simulink model "ME131_lab8"  (R2018b)
settings: Solver=VariableStepAuto  StartTime=0.0  StopTime=29  RelTol=1e-3
undefined symbols (not defined in the file): Cf, Cr, dt, Iz, Lf, Lr, m, Vx0, Vy0, X0, Y0, yaw0, yawRate0
settings Model: Creator=YW_Liao  LastModifiedBy=trey
settings SFSimCC: SimUseLocalCustomCode=off
settings RTWCC: RTWUseLocalCustomCode=off

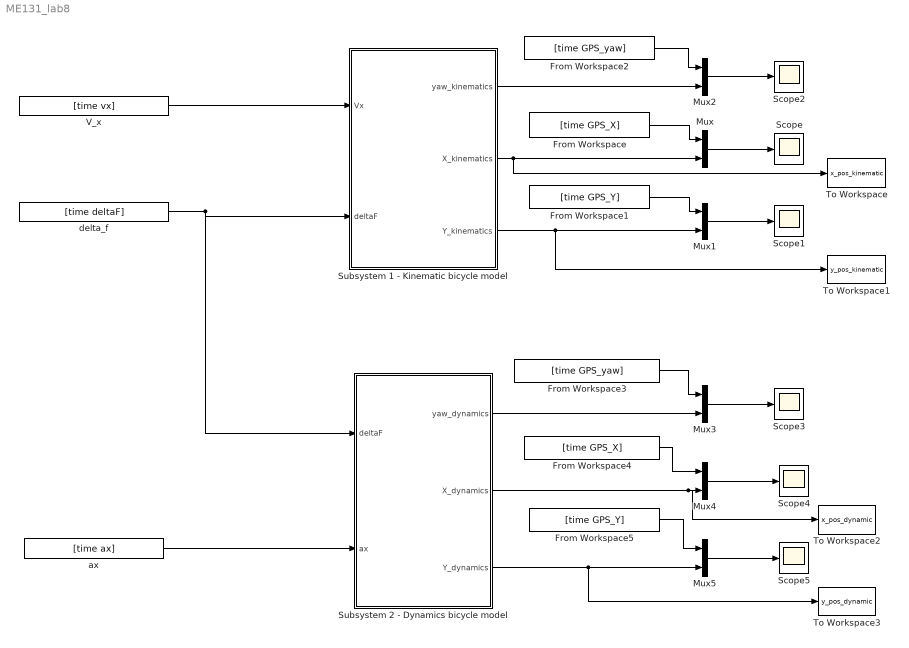
== system ME131_lab8 ==
  From Workspace : FromWorkspace  VariableName=[time GPS_X]  SampleTime=dt
  From Workspace1 : FromWorkspace  VariableName=[time GPS_Y]  SampleTime=dt
  From Workspace2 : FromWorkspace  VariableName=[time GPS_yaw]  SampleTime=dt
  From Workspace3 : FromWorkspace  VariableName=[time GPS_yaw]  SampleTime=dt
  From Workspace4 : FromWorkspace  VariableName=[time GPS_X]  SampleTime=dt
  From Workspace5 : FromWorkspace  VariableName=[time GPS_Y]  SampleTime=dt
  Mux{,1..5} (6 alike) : Mux  Inputs=2
  Scope{,1..5} (6 alike) : Scope
  Subsystem 1 - Kinematic bicycle model : Subsystem
  Subsystem 2 - Dynamics bicycle model : Subsystem
  To Workspace : ToWorkspace  VariableName=x_pos_kinematic  SaveFormat=Timeseries  SampleTime=-1
  To Workspace1 : ToWorkspace  VariableName=y_pos_kinematic  SaveFormat=Timeseries  SampleTime=-1
  To Workspace2 : ToWorkspace  VariableName=x_pos_dynamic  SaveFormat=Timeseries  SampleTime=-1
  To Workspace3 : ToWorkspace  VariableName=y_pos_dynamic  SaveFormat=Timeseries  SampleTime=-1
  V_x : FromWorkspace  VariableName=[time vx]  SampleTime=dt
  ax : FromWorkspace  VariableName=[time ax]  SampleTime=dt
  delta_f : FromWorkspace  VariableName=[time deltaF]  SampleTime=dt
  wires:
  Mux1/1 -> Scope1/1
  Mux/1 -> Scope/1
  From Workspace/1 -> Mux/1
  From Workspace1/1 -> Mux1/1
  Mux2/1 -> Scope2/1
  From Workspace2/1 -> Mux2/1
  From Workspace4/1 -> Mux4/1
  From Workspace3/1 -> Mux3/1
  Mux3/1 -> Scope3/1
  Mux4/1 -> Scope4/1
  Mux5/1 -> Scope5/1
  From Workspace5/1 -> Mux5/1
  Subsystem 1 - Kinematic bicycle model/3(Y_kinematics) -> To Workspace1/1, Mux1/2
  Subsystem 1 - Kinematic bicycle model/2(X_kinematics) -> To Workspace/1, Mux/2
  V_x/1 -> Subsystem 1 - Kinematic bicycle model/1(Vx)
  delta_f/1 -> Subsystem 2 - Dynamics bicycle model/1(deltaF), Subsystem 1 - Kinematic bicycle model/2(deltaF)
  Subsystem 1 - Kinematic bicycle model/1(yaw_kinematics) -> Mux2/2
  ax/1 -> Subsystem 2 - Dynamics bicycle model/2(ax)
  Subsystem 2 - Dynamics bicycle model/1(yaw_dynamics) -> Mux3/2
  Subsystem 2 - Dynamics bicycle model/2(X_dynamics) -> To Workspace2/1, Mux4/2
  Subsystem 2 - Dynamics bicycle model/3(Y_dynamics) -> To Workspace3/1, Mux5/2

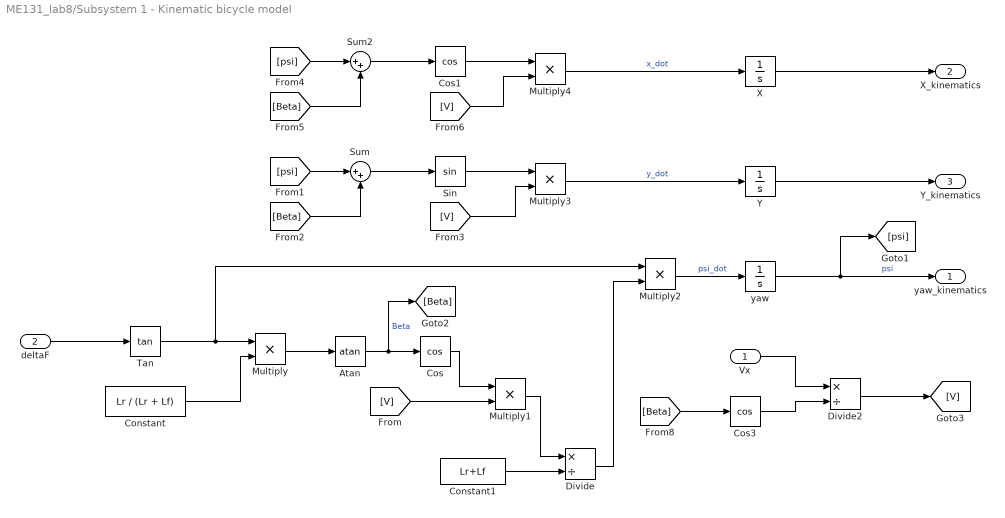
== system ME131_lab8/Subsystem 1 - Kinematic bicycle model ==
  Vx : Inport
  deltaF : Inport  Port=2
  Atan : Trigonometry  Operator=atan
  Constant : Constant  Value=Lr / (Lr + Lf)
  Constant1 : Constant  Value=Lr+Lf
  Cos : Trigonometry  Operator=cos
  Cos1 : Trigonometry  Operator=cos
  Cos3 : Trigonometry  Operator=cos
  Divide : Product  Inputs=*/
  Divide2 : Product  Inputs=*/
  Multiply{,1..4} (5 alike) : Product
  Sin : Trigonometry
  Sum : Sum  Inputs=|++
  Sum2 : Sum  Inputs=|++
  Tan : Trigonometry  Operator=tan
  X : Integrator  InitialCondition=X0
  Y : Integrator  InitialCondition=Y0
  yaw : Integrator  InitialCondition=yaw0
  yaw_kinematics : Outport
  X_kinematics : Outport  Port=2
  Y_kinematics : Outport  Port=3
  wires:
  yaw/1 -> yaw_kinematics/1, [psi]  "psi"
  X/1 -> X_kinematics/1
  Y/1 -> Y_kinematics/1
  deltaF/1 -> Tan/1
  Tan/1 -> Multiply2/1, Multiply/1
  Constant/1 -> Multiply/2
  Multiply/1 -> Atan/1
  Atan/1 -> [Beta], Cos/1  "Beta"
  Constant1/1 -> Divide/2
  Multiply3/1 -> Y/1  "y_dot"
  Cos/1 -> Multiply1/1
  [V] -> Multiply1/2
  Multiply1/1 -> Divide/1
  Divide/1 -> Multiply2/2
  Multiply2/1 -> yaw/1  "psi_dot"
  Sum/1 -> Sin/1
  Sin/1 -> Multiply3/1
  [psi] -> Sum/1
  Vx/1 -> Divide2/1
  [Beta] -> Sum/2
  [V] -> Multiply3/2
  [Beta] -> Sum2/2
  [psi] -> Sum2/1
  Sum2/1 -> Cos1/1
  [V] -> Multiply4/2
  Cos1/1 -> Multiply4/1
  Multiply4/1 -> X/1  "x_dot"
  [Beta] -> Cos3/1
  Cos3/1 -> Divide2/2
  Divide2/1 -> [V]

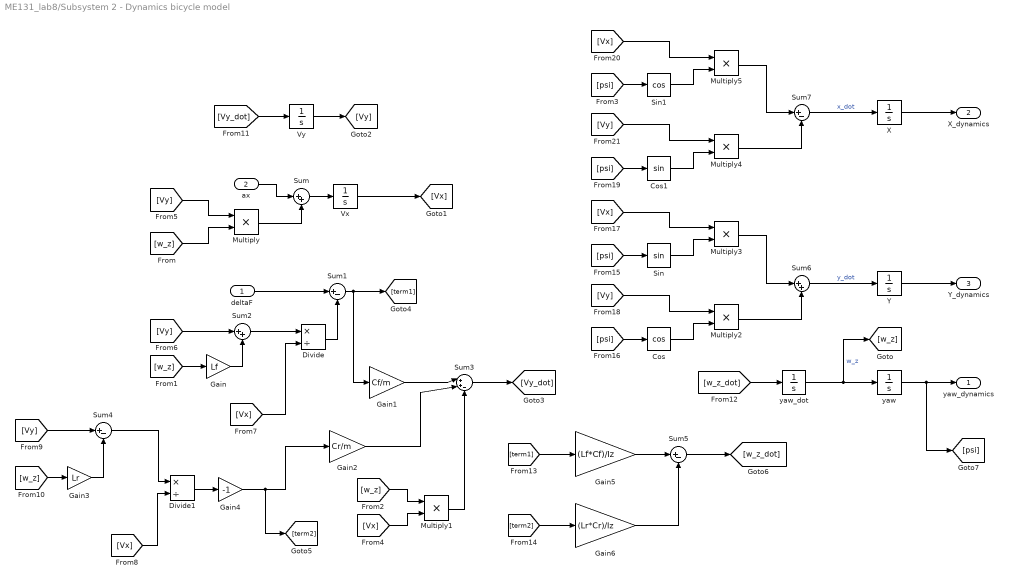
== system ME131_lab8/Subsystem 2 - Dynamics bicycle model ==
  deltaF : Inport
  ax : Inport  Port=2
  Cos : Trigonometry  Operator=cos
  Cos1 : Trigonometry
  Divide : Product  Inputs=*/
  Divide1 : Product  Inputs=*/
  Gain : Gain  Gain=Lf
  Gain1 : Gain  Gain=Cf/m
  Gain2 : Gain  Gain=Cr/m
  Gain3 : Gain  Gain=Lr
  Gain4 : Gain  Gain=-1
  Gain5 : Gain  Gain=(Lf*Cf)/Iz
  Gain6 : Gain  Gain=(Lr*Cr)/Iz
  Multiply{,1..5} (6 alike) : Product
  Sin : Trigonometry
  Sin1 : Trigonometry  Operator=cos
  Sum : Sum  Inputs=|++
  Sum{1,4..5,7} (4 alike) : Sum  Inputs=|+-
  Sum2 : Sum  Inputs=|++
  Sum3 : Sum  Inputs=|++-
  Sum6 : Sum  Inputs=|++
  Vx : Integrator  InitialCondition=Vx0
  Vy : Integrator  InitialCondition=Vy0
  X : Integrator  InitialCondition=X0
  Y : Integrator  InitialCondition=Y0
  yaw : Integrator  InitialCondition=yaw0
  yaw_dot : Integrator  InitialCondition=yawRate0
  yaw_dynamics : Outport
  X_dynamics : Outport  Port=2
  Y_dynamics : Outport  Port=3
  wires:
  Y/1 -> Y_dynamics/1
  yaw_dot/1 -> [w_z], yaw/1  "w_z"
  X/1 -> X_dynamics/1
  yaw/1 -> [psi], yaw_dynamics/1
  Multiply/1 -> Sum/2
  [w_z] -> Multiply/2
  deltaF/1 -> Sum1/1
  [w_z] -> Gain/1
  Gain/1 -> Sum2/2
  Sum2/1 -> Divide/1
  Divide/1 -> Sum1/2
  Sum1/1 -> Gain1/1, [term1]
  Gain1/1 -> Sum3/1
  Multiply1/1 -> Sum3/3
  [w_z] -> Multiply1/1
  [Vx] -> Multiply1/2
  Vy/1 -> [Vy]
  [Vy] -> Multiply/1
  [Vy] -> Sum2/1
  [Vx] -> Divide/2
  Gain2/1 -> Sum3/2
  [Vx] -> Divide1/2
  [w_z] -> Gain3/1
  [Vy] -> Sum4/1
  Gain3/1 -> Sum4/2
  Sum4/1 -> Divide1/1
  Divide1/1 -> Gain4/1
  Sum3/1 -> [Vy_dot]
  [Vy_dot] -> Vy/1
  Gain5/1 -> Sum5/1
  Gain6/1 -> Sum5/2
  Sum5/1 -> [w_z_dot]
  [w_z_dot] -> yaw_dot/1
  [term2] -> Gain6/1
  [term1] -> Gain5/1
  [psi] -> Cos/1
  [psi] -> Sin/1
  Sum6/1 -> Y/1  "y_dot"
  [Vy] -> Multiply2/1
  Cos/1 -> Multiply2/2
  [Vx] -> Multiply3/1
  Sin/1 -> Multiply3/2
  Multiply3/1 -> Sum6/1
  Multiply2/1 -> Sum6/2
  Gain4/1 -> [term2], Gain2/1
  Sum/1 -> Vx/1
  ax/1 -> Sum/1
  Vx/1 -> [Vx]
  Multiply4/1 -> Sum7/2
  Multiply5/1 -> Sum7/1
  Sin1/1 -> Multiply5/2
  [Vx] -> Multiply5/1
  Cos1/1 -> Multiply4/2
  [Vy] -> Multiply4/1
  Sum7/1 -> X/1  "x_dot"
  [psi] -> Sin1/1
  [psi] -> Cos1/1
